simulink model "controlproporcional"  (R2024b)
settings: Solver=VariableStepAuto  StartTime=0.0  StopTime=10.0  RelTol=1e-3
libraries: fuzblock x1
settings Model: Creator=juanp  LastModifiedBy=juanp

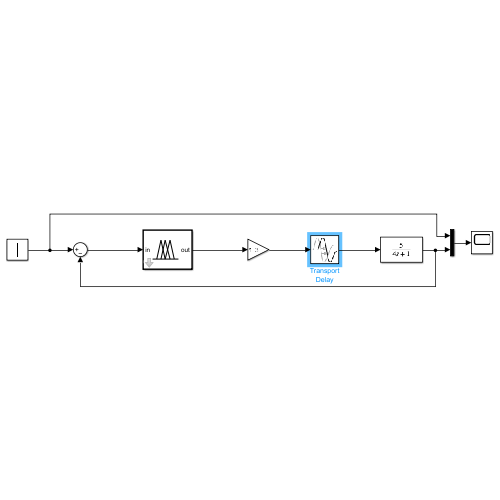
[thumbnail: Simulink's stored preview of the top-level diagram]
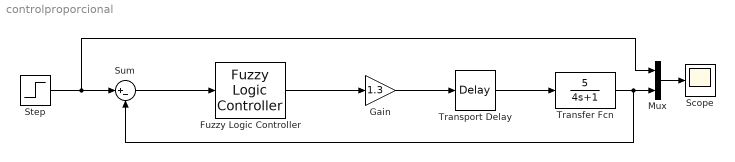
== system controlproporcional ==
  Fuzzy Logic Controller : fuzblock/Fuzzy Logic  Controller  FIS='controlD.fis'  OutputSampleNumber=101  DataType=double  FuzzifiedInputs=off  RuleFiringStrengths=off  RuleOutputs=off  AggregatedOutputs=off  SimulateUsing=Interpreted execution  OutOfRangeInputValueMessage=warning  NoRuleFiredMessage=warning  EmptyOutputFuzzySetMessage=warning
  Gain : Gain  Gain=1.3
  Mux : Mux  Inputs=2
  Scope : Scope
  Step : Step  SampleTime=0
  Sum : Sum  Inputs=|+-
  Transfer Fcn : TransferFcn  Numerator=[5]  Denominator=[4 1]
  Transport Delay : TransportDelay  DelayTime=0.2
  wires:
  Step/1 -> Mux/1, Sum/1
  Fuzzy Logic Controller/1 -> Gain/1
  Sum/1 -> Fuzzy Logic Controller/1
  Gain/1 -> Transport Delay/1
  Transport Delay/1 -> Transfer Fcn/1
  Transfer Fcn/1 -> Sum/2, Mux/2
  Mux/1 -> Scope/1
